simulink model "chap7_6sim"  (Simulink 5.0)
settings: Solver=ode45  StartTime=0.0  StopTime=20.0  RelTol=1e-3
settings Model: LastModifiedBy=Administrator

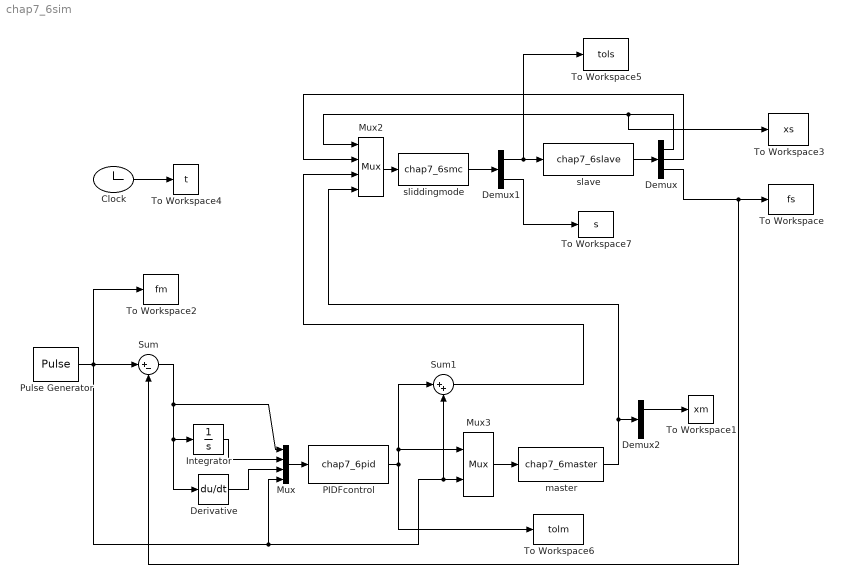
== system chap7_6sim ==
  Clock : Clock
      settings: Decimation=10
  Demux : Demux  Outputs=3
  Demux1 : Demux  Outputs=2
  Demux2 : Demux  Outputs=2
  Derivative : Derivative
  Integrator : Integrator
  Mux : Mux
  Mux2 : Mux
  Mux3 : Mux  Inputs=2
  PIDFcontrol : S-Function  FunctionName=chap7_6pid
  Pulse Generator : DiscretePulseGenerator  PulseType=Time based  Amplitude=50  Period=10  PulseWidth=50
  Sum : Sum  Inputs=|+-  SaturateOnIntegerOverflow=on
  Sum1 : Sum  Inputs=|++  SaturateOnIntegerOverflow=on
  To Workspace : ToWorkspace  VariableName=fs  SampleTime=-1  SaveFormat=Array
  To Workspace1 : ToWorkspace  VariableName=xm  SampleTime=-1  SaveFormat=Array
  To Workspace2 : ToWorkspace  VariableName=fm  SampleTime=-1  SaveFormat=Array
  To Workspace3 : ToWorkspace  VariableName=xs  SampleTime=-1  SaveFormat=Array
  To Workspace4 : ToWorkspace  VariableName=t  SampleTime=-1  SaveFormat=Array
  To Workspace5 : ToWorkspace  VariableName=tols  SampleTime=-1  SaveFormat=Array
  To Workspace6 : ToWorkspace  VariableName=tolm  SampleTime=-1  SaveFormat=Array
  To Workspace7 : ToWorkspace  VariableName=s  SampleTime=-1  SaveFormat=Array
  master : S-Function  FunctionName=chap7_6master
  slave : S-Function  FunctionName=chap7_6slave
  sliddingmode : S-Function  FunctionName=chap7_6smc
  wires:
  Mux2/1 -> sliddingmode/1
  slave/1 -> Demux/1
  Demux/1 -> Mux2/1, To Workspace3/1
  Demux/2 -> Mux2/2
  Demux/3 -> Sum/2, To Workspace/1
  Demux1/1 -> slave/1, To Workspace5/1
  Demux1/2 -> To Workspace7/1
  sliddingmode/1 -> Demux1/1
  master/1 -> Mux2/4, Demux2/1
  PIDFcontrol/1 -> Mux3/1, Sum1/1, To Workspace6/1
  Mux/1 -> PIDFcontrol/1
  Integrator/1 -> Mux/2
  Sum/1 -> Mux/1, Integrator/1, Derivative/1
  Demux2/1 -> To Workspace1/1
  Clock/1 -> To Workspace4/1
  Pulse Generator/1 -> Sum/1, To Workspace2/1, Mux/4, Mux3/2, Sum1/2
  Mux3/1 -> master/1
  Derivative/1 -> Mux/3
  Sum1/1 -> Mux2/3
